simulink library "HDL_ieee_8021513"  (R2024a)
settings: Solver=FixedStepDiscrete  StartTime=0.0  StopTime=10.0  RelTol=1e-3
undefined symbols (not defined in the file): Add, axiWidth, CONST, fs, peakDetectorThreshold, peakDetectorWindow, QAM, Shift
libraries: hdlsllib x199, $bdroot x91, whdlutilities x34, whdledac x9, simulink x8, whdlmod x6, dspsigops x5, dsphdlfiltering2 x4, embreciprocals x3, dsphdlsigops2 x2, commhdlcrc x2, dspstat3 x2
(part 1 of 6)
settings Model: Creator=cotti  LastModifiedBy=cotti
settings OptimizationCC: BlockReduction=off  ConditionallyExecuteInputs=off  DefaultParameterBehavior=Inlined  InheritOutputTypeSmallerThanSingle=on  ReuseModelBlockBuffer=off
settings DebuggingCC: AlgebraicLoopMsg=error  SingleTaskRateTransMsg=error
settings HardwareCC: ProdBitPerPointer=32  ProdBitPerSizeT=32  ProdBitPerPtrDiffT=32  ProdLargestAtomicFloat=None  ProdIntDivRoundTo=Undefined  ProdEndianess=Unspecified  ProdWordSize=32  ProdHWDeviceType=ASIC/FPGA->ASIC/FPGA  TargetBitPerLong=64  TargetBitPerPointer=64  TargetBitPerSizeT=64  TargetBitPerPtrDiffT=64  TargetLongLongMode=on  TargetIntDivRoundTo=Zero  TargetEndianess=LittleEndian  TargetWordSize=64  TargetHWDeviceType=Custom Processor->MATLAB Host Computer  ProdEqTarget=off
settings RTWCC: GPUComputeCapability=3.5

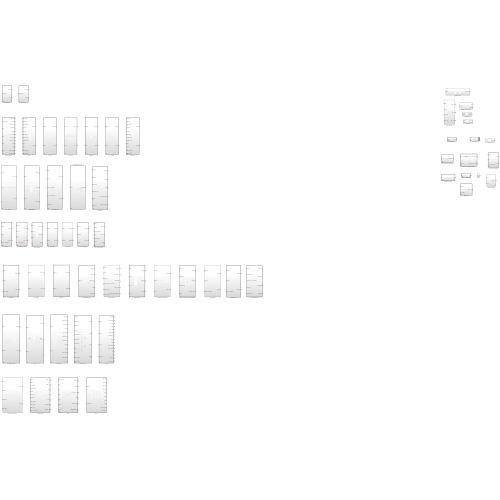
[thumbnail: Simulink's stored preview of the top-level diagram]
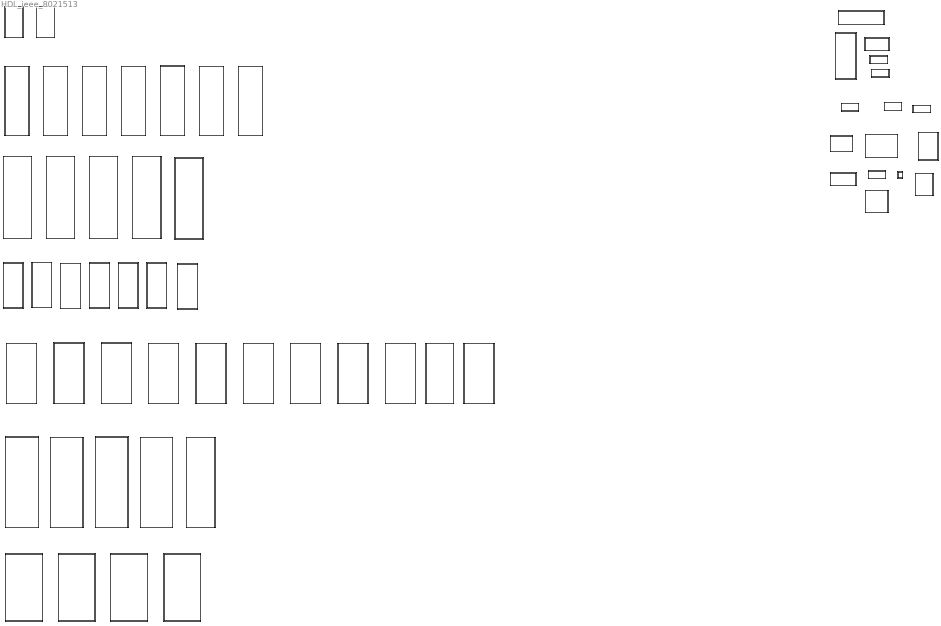
== system HDL_ieee_8021513 ==
  4QAM_demod : Subsystem  TreatAsAtomicUnit=on
  Buffer : Subsystem
  Deco_3a8 : Subsystem
  batid_to_bits_per_subcarrier : Subsystem
  calculate_mean_and_std : Subsystem
  channel_estimation_and_equalization : Subsystem  TreatAsAtomicUnit=on
  channel_gen : Subsystem
  complex_multiplier : Subsystem
  constellation_descrambler : Subsystem
  constellation_scrambler : Subsystem
  decimator : Subsystem  TreatAsAtomicUnit=on
  downshifter : Subsystem  TreatAsAtomicUnit=on
  falling_edge_detector : Subsystem
  frequency_upshift : Subsystem
  full_ofdm_modulator : Subsystem  TreatAsAtomicUnit=on
  full_rx : Subsystem  TreatAsAtomicUnit=on
  full_tx : Subsystem  TreatAsAtomicUnit=on
  gnd_ctrl : Subsystem
  h_crc : Subsystem
  h_crc_rx : Subsystem
  h_gen : Subsystem
  h_remove_repetition : Subsystem
  h_repetition : Subsystem
  h_rx_full : Subsystem  TreatAsAtomicUnit=on
  h_scrambler : Subsystem
      settings: LibrarySourceBlock=|
      | hdlsllib/Ports &
      | Subsystems/Subsystem
  h_separate : Subsystem
  header_fec : Subsystem
  header_full : Subsystem  TreatAsAtomicUnit=on
      settings: LibrarySourceBlock=|
      | hdlsllib/Ports &
      | Subsystems/Subsystem
  interpolator : Subsystem
  ldpc_encoder : Subsystem
  lfsr_const_scrambler : Subsystem
  next_frame_to_ready : Subsystem
  ofdm_demod : Subsystem  TreatAsAtomicUnit=on
  ofdm_modulator : Subsystem
  ofdm_separator : Subsystem
  ofdm_symbol_sync : Subsystem  TreatAsAtomicUnit=on
  p_scrambler : Subsystem
      settings: LibrarySourceBlock=|
      | hdlsllib/Ports &
      | Subsystems/Subsystem
  payload_full : Subsystem  TreatAsAtomicUnit=on
  payload_rep : Subsystem
  peak_detector : Subsystem
  preamble_gen : Subsystem
  psdu_size_to_payload_length : Subsystem
  puncturer : Subsystem
  qam_demod : Subsystem
  qam_mod : Subsystem
  reduced_ldpc : Subsystem
  reg_to_variable : Subsystem
  remove_tone_mapping : Subsystem
  rising_edge_detector : Subsystem
  rx_demodulator_full : Subsystem  TreatAsAtomicUnit=on
  rx_interpolator : Subsystem
  rx_payload_full : Subsystem  TreatAsAtomicUnit=on
  signal_ack : Subsystem
  tone_mapping : Subsystem
  tx_decimator : Subsystem
  valid_to_ctrl : Subsystem
  variable_to_reg : Subsystem

== system HDL_ieee_8021513/4QAM_demod ==
  data_in : Inport
  valid_in : Inport  Port=2
  bits_per_subcarrier : Inport  Port=3
  Delay{,1,3..4} (4 alike) : Delay  DelayLength=1  InitialCondition=0  UseCircularBuffer=on
  Delay2 : Delay  DelayLength=5  InitialCondition=0  UseCircularBuffer=on
  Symbol Demodulator1 : whdlmod/Symbol Demodulator  ModulationSource=Property  ModulationScheme=QPSK  MaxModulation=256-QAM  ConstOrder=Default  ConstMap=[ 2, 3, 1, 0, 6, 7, 5, 4, 14, 15, 13, 12, 10, 11, 9, 8 ]  DecisionType=Approximate log-likelihood ratio  PhaseOffset=-pi/4  OutputType=Vector  NormMethod=Unit average power  MinSymDistance=2  NoiseVariance=off  SimulateUsing=Code generation
  Terminator : Terminator
  Terminator2 : Terminator
  convert_with_rounding : DataTypeConversion  OutDataTypeStr=CONST.rxQAMDemodDataType  RndMeth=Round  SaturateOnIntegerOverflow=off
  data_out : Outport
  valid_out : Outport  Port=2  VectorParamsAs1DForOutWhenUnconnected=off
  wires:
  Delay4/1 -> Delay1/1
  Delay3/1 -> convert_with_rounding/1
  convert_with_rounding/1 -> Delay/1
  Symbol Demodulator1/2 -> Terminator2/1
  data_in/1 -> Symbol Demodulator1/1
  Symbol Demodulator1/1 -> Delay3/1
  valid_in/1 -> Symbol Demodulator1/2, Delay2/1
  Delay1/1 -> valid_out/1
  Delay/1 -> data_out/1
  bits_per_subcarrier/1 -> Terminator/1
  Delay2/1 -> Delay4/1

== system HDL_ieee_8021513/Buffer ==
  I : Inport
  O : Outport
  wires:
  I/1 -> O/1

== system HDL_ieee_8021513/Deco_3a8 ==
  in0 : Inport
  in1 : Inport  Port=2
  in2 : Inport  Port=3
  Logical Operator{,1..7} (8 alike) : Logic  Inputs=3  IconShape=distinctive  AllPortsSameDT=off  OutDataTypeStr=boolean
  Logical Operator{8..11,13..15,17,21..22,25,27} (12 alike) : Logic  Operator=NOT  IconShape=distinctive  AllPortsSameDT=off  OutDataTypeStr=boolean
  m0 : Outport
  m1 : Outport  Port=2
  m2 : Outport  Port=3
  m3 : Outport  Port=4
  m4 : Outport  Port=5
  m5 : Outport  Port=6
  m6 : Outport  Port=7
  m7 : Outport  Port=8
  wires:
  Logical Operator/1 -> m0/1
  Logical Operator1/1 -> m1/1
  Logical Operator2/1 -> m2/1
  Logical Operator3/1 -> m3/1
  Logical Operator4/1 -> m4/1
  Logical Operator5/1 -> m5/1
  Logical Operator6/1 -> m6/1
  Logical Operator7/1 -> m7/1
  in0/1 -> [in0]
  in1/1 -> [in1]
  in2/1 -> [in2]
  [in0] -> Logical Operator8/1
  [in1] -> Logical Operator9/1
  [in2] -> Logical Operator10/1
  Logical Operator8/1 -> Logical Operator/1
  Logical Operator9/1 -> Logical Operator/2
  Logical Operator10/1 -> Logical Operator/3
  [in1] -> Logical Operator13/1
  [in2] -> Logical Operator11/1
  [in2] -> Logical Operator14/1
  [in0] -> Logical Operator15/1
  [in1] -> Logical Operator2/2
  [in2] -> Logical Operator17/1
  [in0] -> Logical Operator3/1
  [in1] -> Logical Operator3/2
  [in2] -> Logical Operator4/3
  [in0] -> Logical Operator21/1
  [in1] -> Logical Operator22/1
  [in2] -> Logical Operator5/3
  [in0] -> Logical Operator5/1
  [in1] -> Logical Operator25/1
  [in2] -> Logical Operator6/3
  [in0] -> Logical Operator27/1
  [in1] -> Logical Operator6/2
  [in2] -> Logical Operator7/3
  [in0] -> Logical Operator7/1
  [in1] -> Logical Operator7/2
  [in0] -> Logical Operator1/1
  Logical Operator13/1 -> Logical Operator1/2
  Logical Operator11/1 -> Logical Operator1/3
  Logical Operator15/1 -> Logical Operator2/1
  Logical Operator14/1 -> Logical Operator2/3
  Logical Operator22/1 -> Logical Operator4/2
  Logical Operator21/1 -> Logical Operator4/1
  Logical Operator17/1 -> Logical Operator3/3
  Logical Operator27/1 -> Logical Operator6/1
  Logical Operator25/1 -> Logical Operator5/2

== system HDL_ieee_8021513/batid_to_bits_per_subcarrier ==
  note: De momento, el valor de BATID va a coincidir con el valor de la cantidad de bits por subcarrier.
  note: Remember that "bat_id" is LSB first.
  bat_id : Inport
  Bit Concat : hdlsllib/Logic and Bit Operations/Bit Concat  numInputs=4
  Demux : Demux  Outputs=5
  State Control : StateControl  StateControl=Synchronous
  Terminator : Terminator
  bits_per_subcarrier : Outport
  wires:
  bat_id/1 -> Demux/1
  Demux/3 -> [bat2]
  Demux/2 -> [bat1]
  Demux/4 -> [bat3]
  Demux/5 -> Terminator/1
  Demux/1 -> [bat0]
  Bit Concat/1 -> bits_per_subcarrier/1
  [bat3] -> Bit Concat/1
  [bat2] -> Bit Concat/2
  [bat1] -> Bit Concat/3
  [bat0] -> Bit Concat/4

== system HDL_ieee_8021513/calculate_mean_and_std ==
  data_in : Inport
  Delay{6..8,10..11} (5 alike) : Delay  DelayLength=1  InitialCondition=0  UseCircularBuffer=on
  Square : Math  Operator=square  SignedPower=on  RndMeth=Zero
  Subtract : Sum  Inputs=+-  OutDataTypeStr=Inherit: Same as first input
  calculate_mean_x : Subsystem
  calculate_mean_x_squared : Subsystem
  multiply by 2 : hdlsllib/Logic and Bit Operations/Bit Shift  mode=Shift Left Logical  N=1
  std : Outport
  mean : Outport  Port=2
  wires:
  Delay11/1 -> mean/1
  Subtract/1 -> Delay8/1
  Delay10/1 -> Delay11/1
  Square/1 -> Delay7/1
  Delay8/1 -> multiply by 2/1
  Delay6/1 -> Subtract/1
  calculate_mean_x/1(mean) -> Delay10/1, Square/1
  Delay7/1 -> Subtract/2
  calculate_mean_x_squared/1(mean_x_squared) -> Delay6/1
  data_in/1 -> calculate_mean_x/1(data_in), calculate_mean_x_squared/1(data_in)
  multiply by 2/1 -> std/1

== system HDL_ieee_8021513/channel_estimation_and_equalization ==
  note: Stores the estimate from Channel Estimation subsystem for each frame and perform channel equalization.
  note: Estimates the channel frequency response for each frame.
  data_in : Inport
  valid_data : Inport  Port=2
  valid_channel : Inport  Port=3
  reset : Inport  Port=4
  Channel Equalization : Subsystem
  Channel Estimation : Subsystem
  Delay{1..6,10..11,13..14} (10 alike) : Delay  DelayLength=1  InitialCondition=0
  Delay21 : Delay  InitialCondition=0
  Delay22 : Delay  InitialCondition=0
  data_out : Outport
  valid_out : Outport  Port=2
  channel_est_out : Outport  Port=3
  wires:
  reset/1 -> Channel Estimation/3(reset)
  Delay4/1 -> channel_est_out/1
  Channel Equalization/3(channel_est_out) -> Delay4/1
  Channel Estimation/1(channel_estimate) -> Delay13/1  "channelEstimates"
  Delay22/1 -> Delay11/1
  Delay21/1 -> Delay10/1
  valid_channel/1 -> Delay2/1
  data_in/1 -> Delay1/1
  valid_data/1 -> Delay3/1
  Delay2/1 -> Channel Estimation/2(valid_in)
  Channel Estimation/2(valid_estimate) -> Delay14/1  "channelEstimatesValid"
  Delay3/1 -> Delay22/1
  Delay1/1 -> Channel Estimation/1(data_in), Delay21/1
  Channel Equalization/2(valid_out) -> Delay6/1
  Channel Equalization/1(data_out) -> Delay5/1
  Delay10/1 -> Channel Equalization/1(data_in)
  Delay11/1 -> Channel Equalization/2(valid_data)
  Delay13/1 -> Channel Equalization/3(channel_estimate_in)
  Delay14/1 -> Channel Equalization/4(valid_channel_estimate)
  Delay6/1 -> valid_out/1
  Delay5/1 -> data_out/1

== system HDL_ieee_8021513/channel_gen ==
  new_frame : Inport
  Delay : Delay  DelayLength=1  InitialCondition=0  UseCircularBuffer=on
  Direct Lookup Table (n-D) : LookupNDDirect  NumberOfTableDimensions=1  Table=CONST.channelLUT  DiagnosticForOutOfRangeInput=Error  RemoveProtectionInput=on  TableDataTypeStr=boolean
  HDL Counter : hdlsllib/Sources/HDL Counter  CountType=Count limited  CountInit=0  CountStep=1  CountMax=length(CONST.channelLUT)-1  CountFromType=Initial value  CountFrom=0  CountResetPort=off  CountLoadPort=off  CountEnbPort=on  CountDirPort=off  CountHitOutputPort=on  CountDataType=Unsigned  CountWordLen=nextpow2(length(CONST.channelLUT))  CountFracLen=0  CountSampTime=1
  Logical Operator : Logic  Operator=NOT  IconShape=distinctive  AllPortsSameDT=off  OutDataTypeStr=boolean
  Logical Operator1 : Logic  Operator=OR  IconShape=distinctive  AllPortsSameDT=off  OutDataTypeStr=boolean
  State Control : StateControl  StateControl=Synchronous
  Unit Delay Enabled Synchronous : hdlsllib/Discrete/Unit Delay Enabled Synchronous  InitialCondition=0.0  SampleTime=-1
  valid_to_ctrl : $bdroot/valid_to_ctrl  SystemSampleTime=-1  VariantActivationTime=update diagram  AllowFlexibleInterface=on  Latency=0  AutoFrameSizeCalculation=off
  data_out : Outport
  ctrl_out : Outport  Port=2
  wires:
  Unit Delay Enabled Synchronous/1 -> HDL Counter/1, valid_to_ctrl/1
  HDL Counter/1 -> Direct Lookup Table (n-D)/1
  Logical Operator/1 -> Unit Delay Enabled Synchronous/1
  Direct Lookup Table (n-D)/1 -> Delay/1
  valid_to_ctrl/1 -> ctrl_out/1
  Delay/1 -> data_out/1
  new_frame/1 -> Logical Operator1/1
  HDL Counter/2 -> Logical Operator1/2, Logical Operator/1
  Logical Operator1/1 -> Unit Delay Enabled Synchronous/2

== system HDL_ieee_8021513/complex_multiplier ==
  in_a : Inport
  in_b : Inport  Port=2
  Add : Sum
  Add1 : Sum
  Add2 : Sum
  Complex to Real-Imag1 : ComplexToRealImag
  Complex to Real-Imag2 : ComplexToRealImag
  Delay{,1..3,10} (5 alike) : Delay  DelayLength=1  InitialCondition=0  UseCircularBuffer=on
  Delay{4..9,11,13..14} (9 alike) : Delay  InitialCondition=0  UseCircularBuffer=on
  Product : Product
  Product1 : Product
  Product2 : Product
  Real-Imag to Complex : RealImagToComplex
  Subtract : Sum  Inputs=+-
  Subtract1 : Sum  Inputs=+-
  a_times_b : Outport
  wires:
  [xr] -> Delay7/1
  [yi] -> Delay9/1
  [xi] -> Delay14/1
  [yi] -> Add/2
  [yr] -> Add/1
  [xi] -> Subtract1/2
  [xr] -> Subtract1/1
  [yi] -> Subtract/2
  [yr] -> Subtract/1
  in_a/1 -> Complex to Real-Imag1/1
  Complex to Real-Imag1/1 -> Delay/1
  in_b/1 -> Complex to Real-Imag2/1
  Complex to Real-Imag2/1 -> Delay2/1
  Complex to Real-Imag1/2 -> Delay1/1
  Complex to Real-Imag2/2 -> Delay3/1
  Delay10/1 -> a_times_b/1
  Subtract1/1 -> Delay4/1
  Subtract/1 -> Delay5/1
  Add/1 -> Delay6/1
  Delay4/1 -> Product/1
  Product/1 -> Delay8/1
  Delay/1 -> [xr]
  Delay1/1 -> [xi]
  Delay2/1 -> [yr]
  Delay3/1 -> [yi]
  Delay9/1 -> Product/2
  Delay5/1 -> Product1/1
  Delay7/1 -> Product1/2
  Product1/1 -> Delay11/1
  Add1/1 -> Real-Imag to Complex/1
  Real-Imag to Complex/1 -> Delay10/1
  Product2/1 -> Delay13/1
  Delay6/1 -> Product2/1
  Delay14/1 -> Product2/2
  Delay13/1 -> Add2/2
  Delay11/1 -> Add1/1
  Delay8/1 -> Add2/1, Add1/2
  Add2/1 -> Real-Imag to Complex/2

== system HDL_ieee_8021513/constellation_descrambler ==
  data_in : Inport
  valid_in : Inport  Port=2
  init : Inport  Port=3
  rising_edge_detector : $bdroot/rising_edge_detector  SystemSampleTime=-1  VariantActivationTime=update diagram  AllowFlexibleInterface=on  Latency=0  AutoFrameSizeCalculation=off
  rotate_-90 : Subsystem
  sync_constellation_scrambler : $bdroot/sync_constellation_scrambler  SystemSampleTime=-1  VariantActivationTime=update diagram  AllowFlexibleInterface=on  Latency=0  AutoFrameSizeCalculation=off
  data_out : Outport
  valid_out : Outport  Port=2
  wires:
  rising_edge_detector/1 -> sync_constellation_scrambler/3  "start"
  rotate_-90/1(data_out) -> data_out/1
  rotate_-90/2(valid_out) -> valid_out/1
  sync_constellation_scrambler/2 -> rotate_-90/4(s2_in)  "s2"
  sync_constellation_scrambler/1 -> rotate_-90/3(s1_in)  "s1"
  valid_in/1 -> rising_edge_detector/1, sync_constellation_scrambler/1, rotate_-90/2(valid_in)  "valid"
  init/1 -> sync_constellation_scrambler/2
  data_in/1 -> rotate_-90/1(data_in)

== system HDL_ieee_8021513/constellation_scrambler ==
  data_in : Inport
  valid_in : Inport  Port=2
  init : Inport  Port=3
  new_ofdm_symbol : Inport  Port=4
  Delay{,1..8} (9 alike) : Delay  DelayLength=1  InitialCondition=0  UseCircularBuffer=on
  Logical Operator : Logic  Operator=OR  IconShape=distinctive  AllPortsSameDT=off  OutDataTypeStr=boolean
  State Control : StateControl  StateControl=Synchronous
  lfsr_const_scrambler : $bdroot/lfsr_const_scrambler  SystemSampleTime=-1  VariantActivationTime=update diagram  AllowFlexibleInterface=on  Latency=0  AutoFrameSizeCalculation=off
  rotate : Subsystem
  data_out : Outport  VectorParamsAs1DForOutWhenUnconnected=off
  valid_out : Outport  Port=2  VectorParamsAs1DForOutWhenUnconnected=off
  wires:
  Delay1/1 -> rotate/2(valid_in)
  Delay/1 -> rotate/1(data_in)
  rotate/2(valid_out) -> Delay3/1
  Delay8/1 -> Delay1/1
  Delay4/1 -> rotate/3(s1)
  new_ofdm_symbol/1 -> lfsr_const_scrambler/3
  init/1 -> lfsr_const_scrambler/2
  Logical Operator/1 -> lfsr_const_scrambler/1
  Delay5/1 -> rotate/4(s2)
  Delay6/1 -> Logical Operator/2
  lfsr_const_scrambler/1 -> Delay4/1
  lfsr_const_scrambler/2 -> Delay5/1
  valid_in/1 -> Logical Operator/1, Delay6/1, Delay8/1  "en"
  data_in/1 -> Delay7/1
  Delay7/1 -> Delay/1  "data_in"
  rotate/1(data_out) -> Delay2/1  "data_out"
  Delay2/1 -> data_out/1  "data_out"
  Delay3/1 -> valid_out/1

== system HDL_ieee_8021513/decimator ==
  note: The data out from this blocks is "valid" one sample, and invalid four samples.
      | This blocks makes sure that the data is valid the five cycles.
      | What happens is that the ZOH might sample the signal when is valid or invalid.
  data_in : Inport
  valid_in : Inport  Port=2
  Delay{,1..2,5,8..11} (8 alike) : Delay  DelayLength=1  InitialCondition=0  UseCircularBuffer=on
  Delay3 : Delay  DelayLength=(CONST.rxDecimatorDelay+2)*3  InitialCondition=0  UseCircularBuffer=on
  Delay4 : Delay  DelayLength=CONST.rxDecimatorDelay/CONST.rxM  InitialCondition=0  UseCircularBuffer=on
  Downsample : DownSample  N=CONST.rxM  RateOptions=Allow multirate processing
  Downsample1 : DownSample  N=CONST.rxM  RateOptions=Allow multirate processing
  FIR Decimator : dsphdlfiltering2/FIR Decimator  Numerator=CONST.rxDecimatorFilter.Numerator  FilterStructure=Direct form systolic  DecimationFactor=CONST.rxM  NumCycles=1  SimulateUsing=Code generation  roundingMode=Floor  overflowMode=off  CoefficientsDataTypeStr=CONST.rxDecimatorCoefficientsDataType  OutputDataTypeStr=CONST.rxDecimatorOutputDataType  ResetInputPort=on  HDLGlobalReset=on
  Logical Operator : Logic  Operator=OR  IconShape=distinctive  AllPortsSameDT=off  OutDataTypeStr=boolean
  Logical Operator1 : Logic  Operator=OR  AllPortsSameDT=off  OutDataTypeStr=boolean
  Logical Operator2 : Logic  IconShape=distinctive  AllPortsSameDT=off  OutDataTypeStr=boolean
  Logical Operator3 : Logic  IconShape=distinctive  AllPortsSameDT=off  OutDataTypeStr=boolean
  Logical Operator4 : Logic  Operator=NOT  IconShape=distinctive  AllPortsSameDT=off  OutDataTypeStr=boolean
  Switch : Switch  Criteria=u2 ~= 0  SaturateOnIntegerOverflow=off  InputSameDT=off
  Unit Delay : UnitDelay  SampleTime=-1  HasFrameUpgradeWarning=on
  falling_edge_detector : $bdroot/falling_edge_detector  SystemSampleTime=-1  VariantActivationTime=update diagram  AllowFlexibleInterface=on  Latency=0  AutoFrameSizeCalculation=off
  rising_edge_detector : $bdroot/rising_edge_detector  SystemSampleTime=-1  VariantActivationTime=update diagram  AllowFlexibleInterface=on  Latency=0  AutoFrameSizeCalculation=off
  data_out : Outport
  valid_out : Outport  Port=2
  wires:
  Unit Delay/1 -> Switch/3
  Delay11/1 -> Logical Operator1/1
  Delay1/1 -> Logical Operator/1, Delay3/1
  Downsample1/1 -> Delay2/1  "data_after_down"
  Delay10/1 -> Delay5/1
  valid_in/1 -> Delay1/1, rising_edge_detector/1
  Delay3/1 -> Logical Operator/2
  falling_edge_detector/1 -> Logical Operator4/1
  FIR Decimator/1 -> Switch/1  "data_out"
  data_in/1 -> Delay10/1  "data_in"
  Delay9/1 -> data_out/1
  Delay5/1 -> FIR Decimator/1
  Logical Operator1/1 -> Downsample/1
  FIR Decimator/2 -> Switch/2, Delay11/1, Logical Operator1/2  "valid_out"
  Downsample/1 -> Delay8/1  "valid_after_down"
  Delay/1 -> Logical Operator3/1
  Delay4/1 -> Logical Operator2/2
  rising_edge_detector/1 -> FIR Decimator/3
  Logical Operator3/1 -> valid_out/1
  Delay2/1 -> Delay9/1
  Logical Operator4/1 -> Logical Operator3/2
  Logical Operator2/1 -> Delay/1, falling_edge_detector/1
  Logical Operator/1 -> FIR Decimator/2
  Delay8/1 -> Logical Operator2/1, Delay4/1
  Switch/1 -> Downsample1/1, Unit Delay/1

== system HDL_ieee_8021513/downshifter ==
  data_in : Inport
  valid_in : Inport  Port=2
  phase_offset : Inport  Port=3
  Add : Sum  OutDataTypeStr=Inherit: Same as first input
  Constant : Constant  Value=2^(CONST.ncoWordLength-2)  OutDataTypeStr=fixdt(0,CONST.ncoWordLength, 0)  SampleTime=1/CONST.fADC
  Constant1 : Constant  Value=fi(2^(CONST.ncoWordLength-1)/CONST.preambleFirstPartOFDMSamples, 0, CONST.rxFreqOffsetWordLength, CONST.rxFreqOffsetFractionLength)  OutDataTypeStr=fixdt(0, CONST.rxFreqOffsetWordLength, CONST.rxFreqOffsetFractionLength)  SampleTime=-1
  Delay : Delay  DelayLength=6  InitialCondition=0  UseCircularBuffer=on
  Delay1 : Delay  DelayLength=4  InitialCondition=0  UseCircularBuffer=on
  Delay{2..3,5,7..12} (9 alike) : Delay  InitialCondition=0  UseCircularBuffer=on
  Delay4 : Delay  DelayLength=1  InitialCondition=0  UseCircularBuffer=on
  NCO : dsphdlsigops2/NCO  PhaseIncrementSource=Input port  PhaseIncrement=ncoPhaseIncrement  PhaseOffsetSource=Property  PhaseOffset=0  DitherSource=None  NumDitherBits=1  SamplesPerFrame=1  LUTCompress=off  ResetAction=on  Waveform=Complex exponential  PhasePort=off  SimulateUsing=Code generation  AccumulatorWL=CONST.ncoWordLength  PhaseQuantization=on  NumQuantizerAccumulatorBits=CONST.ncoQuantization  OutputDataType=Binary point scaling  OutputWL=CONST.rxNCOWordLength  OutputFL=CONST.rxNCOFractionLength
  Product : Product  OutDataTypeStr=int16
  digital_carrier_receiver : Subsystem
  rising_edge_detector : $bdroot/rising_edge_detector  SystemSampleTime=-1  VariantActivationTime=update diagram  AllowFlexibleInterface=on  Latency=0  AutoFrameSizeCalculation=off
  data_out : Outport  VectorParamsAs1DForOutWhenUnconnected=off
  valid_out : Outport  Port=2  VectorParamsAs1DForOutWhenUnconnected=off
  wires:
  Constant1/1 -> Product/2
  Delay12/1 -> Delay7/1
  Delay11/1 -> Delay8/1
  Constant/1 -> Add/1
  Delay10/1 -> Add/2
  Delay9/1 -> Product/1
  Product/1 -> Delay10/1
  Delay4/1 -> rising_edge_detector/1
  valid_in/1 -> Delay12/1
  Delay1/1 -> valid_out/1
  NCO/2 -> Delay1/1
  Delay3/1 -> Delay/1
  digital_carrier_receiver/1(data_out) -> data_out/1
  NCO/1 -> digital_carrier_receiver/2(ncoIn)
  Delay/1 -> digital_carrier_receiver/1(dataIn)
  data_in/1 -> Delay11/1
  Delay2/1 -> NCO/3  "valid"
  rising_edge_detector/1 -> NCO/2
  Delay5/1 -> NCO/1  "inc"
  Add/1 -> Delay5/1
  Delay7/1 -> Delay2/1, Delay4/1
  Delay8/1 -> Delay3/1
  phase_offset/1 -> Delay9/1

== system HDL_ieee_8021513/falling_edge_detector ==
  in : Inport
  Delay : Delay  DelayLength=1  InitialCondition=0  UseCircularBuffer=on
  Logical Operator : Logic  IconShape=distinctive  AllPortsSameDT=off  OutDataTypeStr=boolean
  Logical Operator1 : Logic  Operator=NOT  IconShape=distinctive  AllPortsSameDT=off  OutDataTypeStr=boolean
  State Control : StateControl  StateControl=Synchronous
  out : Outport  VectorParamsAs1DForOutWhenUnconnected=off
  wires:
  in/1 -> Logical Operator1/1, Delay/1
  Delay/1 -> Logical Operator/2
  Logical Operator/1 -> out/1
  Logical Operator1/1 -> Logical Operator/1

== system HDL_ieee_8021513/frequency_upshift ==
  data_in : Inport
  valid_in : Inport  Port=2
  reset : Inport  Port=3
  Data Type Conversion : DataTypeConversion  OutDataTypeStr=CONST.ipCoreDataType  SaturateOnIntegerOverflow=off  RndMeth=Floor
  Delay : Delay  DelayLength=6  InitialCondition=0  UseCircularBuffer=on
  Delay1 : Delay  DelayLength=12  InitialCondition=0  UseCircularBuffer=on
  Delay2 : Delay  DelayLength=1  InitialCondition=0  UseCircularBuffer=on
  Delay3 : Delay  DelayLength=1  InitialCondition=0  UseCircularBuffer=on
  Mixer : Subsystem
  NCO : dsphdlsigops2/NCO  PhaseIncrementSource=Property  PhaseIncrement=CONST.ncoUpCarrierPhaseIncrement  PhaseOffsetSource=Property  PhaseOffset=0  DitherSource=None  NumDitherBits=1  SamplesPerFrame=1  LUTCompress=off  ResetAction=on  Waveform=Complex exponential  PhasePort=off  SimulateUsing=Code generation  AccumulatorWL=CONST.ncoUpWordLength  PhaseQuantization=on  NumQuantizerAccumulatorBits=CONST.ncoUpQuantization  OutputDataType=Binary point scaling  OutputWL=CONST.txNCOWordLength  OutputFL=CONST.txNCOFractionLength
  State Control : StateControl  StateControl=Synchronous
  data_out : Outport  VectorParamsAs1DForOutWhenUnconnected=off
  valid_out : Outport  Port=2  VectorParamsAs1DForOutWhenUnconnected=off
  wires:
  Data Type Conversion/1 -> data_out/1
  Delay2/1 -> NCO/2
  reset/1 -> NCO/1
  Delay3/1 -> Delay/1
  data_in/1 -> Delay3/1
  valid_in/1 -> Delay2/1
  NCO/1 -> Mixer/2(ncoIn)
  Mixer/1(mixedOut) -> Data Type Conversion/1
  Delay/1 -> Mixer/1(dataIn)
  NCO/2 -> Delay1/1
  Delay1/1 -> valid_out/1

== system HDL_ieee_8021513/full_ofdm_modulator ==
  data_in : Inport
  valid_in : Inport  Port=2
  bits_per_subcarrier : Inport  Port=3
  init : Inport  Port=4
  new_ofdm_sym : Inport  Port=5
  cp_len : Inport  Port=6
  rst : Inport  Port=7
  Constant : Constant  Value=0  OutDataTypeStr=fixdt(1,16,14)  SampleTime=-1
  Delay{,1,4..11} (10 alike) : Delay  DelayLength=1  InitialCondition=0  UseCircularBuffer=on
  HDL FIFO : hdlsllib/HDL RAMs/HDL FIFO  fifo_size=CONST.preambleFirstPartOFDMSamples  mode=Classic  ratio=1  push_msg=Error  pop_msg=Error  show_empty=on  show_full=on  show_num=off  LabelModeActiveChoice_Mode=Classic  rst_port=on
  Logical Operator1 : Logic  Operator=OR  AllPortsSameDT=off  OutDataTypeStr=boolean
  Real-Imag to Complex : RealImagToComplex
  Repeat : dspsigops/Repeat  FactorSource=Dialog parameter  N=CONST.txL  Nmax=16  RateOptions=Allow multirate processing  ic=0  mode=Unused parameter value
      settings: LibrarySourceBlock=dsphdlsupportsigops/Repeat
  State Control : StateControl  StateControl=Synchronous
  Switch : Switch  Criteria=u2 ~= 0  SaturateOnIntegerOverflow=off  InputSameDT=off
  Switch1 : Switch  Criteria=u2 ~= 0  SaturateOnIntegerOverflow=off  InputSameDT=off
  Unit Delay : UnitDelay  SampleTime=-1  HasFrameUpgradeWarning=on
  constellation_scrambler : $bdroot/constellation_scrambler  SystemSampleTime=-1  VariantActivationTime=update diagram  AllowFlexibleInterface=on  Latency=0  AutoFrameSizeCalculation=off
  frequency_upshift : $bdroot/frequency_upshift  SystemSampleTime=-1  VariantActivationTime=update diagram  AllowFlexibleInterface=on  Latency=0  AutoFrameSizeCalculation=off
  interpolator : $bdroot/interpolator  SystemSampleTime=-1  VariantActivationTime=update diagram  AllowFlexibleInterface=on  Latency=0  AutoFrameSizeCalculation=off
  ofdm_modulator : $bdroot/ofdm_modulator  SystemSampleTime=-1  VariantActivationTime=update diagram  AllowFlexibleInterface=on  Latency=0  AutoFrameSizeCalculation=off
  ofdm_ready_truncate : Subsystem
  qam_mod : $bdroot/qam_mod  SystemSampleTime=-1  VariantActivationTime=update diagram  AllowFlexibleInterface=on  Latency=0  AutoFrameSizeCalculation=off
  data_out : Outport  VectorParamsAs1DForOutWhenUnconnected=off
  valid_out : Outport  Port=2  VectorParamsAs1DForOutWhenUnconnected=off
  ready : Outport  Port=3  VectorParamsAs1DForOutWhenUnconnected=off
  wires:
  Constant/1 -> Real-Imag to Complex/1, Real-Imag to Complex/2
  Real-Imag to Complex/1 -> Switch1/3
  HDL FIFO/1 -> Switch1/1  "fifo_out"
  Switch1/1 -> interpolator/1
  ofdm_modulator/3 -> ofdm_ready_truncate/1(next_frame)  "ready_out"
  Delay10/1 -> qam_mod/2  "real_valid"
  Delay11/1 -> qam_mod/1
  Delay9/1 -> qam_mod/3
  Delay8/1 -> Delay/1
  Delay7/1 -> Delay1/1
  Delay5/1 -> ofdm_modulator/4, HDL FIFO/4, Repeat/1, ofdm_ready_truncate/2(new_psdu)  "fifo_rst"
  ofdm_ready_truncate/1(ready) -> ready/1  "ready"
  Repeat/1 -> frequency_upshift/3
  Delay4/1 -> interpolator/2, Switch1/2
  HDL FIFO/2 -> Logical Operator1/2  "fifo_empty"
  Logical Operator1/1 -> Switch/2
  Switch/1 -> HDL FIFO/3, Unit Delay/1, Delay4/1
  HDL FIFO/3 -> Logical Operator1/1, Switch/1
  Unit Delay/1 -> Switch/3
  ofdm_modulator/1 -> HDL FIFO/1
  ofdm_modulator/2 -> HDL FIFO/2
  rst/1 -> Delay5/1
  Delay1/1 -> constellation_scrambler/4
  Delay/1 -> constellation_scrambler/3
  qam_mod/2 -> constellation_scrambler/2
  qam_mod/1 -> constellation_scrambler/1
  new_ofdm_sym/1 -> Delay7/1
  constellation_scrambler/1 -> ofdm_modulator/1  "out_new"
  constellation_scrambler/2 -> ofdm_modulator/2  "valid_new"
  data_in/1 -> Delay11/1
  valid_in/1 -> Delay10/1
  bits_per_subcarrier/1 -> Delay9/1
  init/1 -> Delay8/1
  cp_len/1 -> Delay6/1
  Delay6/1 -> ofdm_modulator/3
  interpolator/2 -> frequency_upshift/2
  interpolator/1 -> frequency_upshift/1
  frequency_upshift/2 -> valid_out/1
  frequency_upshift/1 -> data_out/1

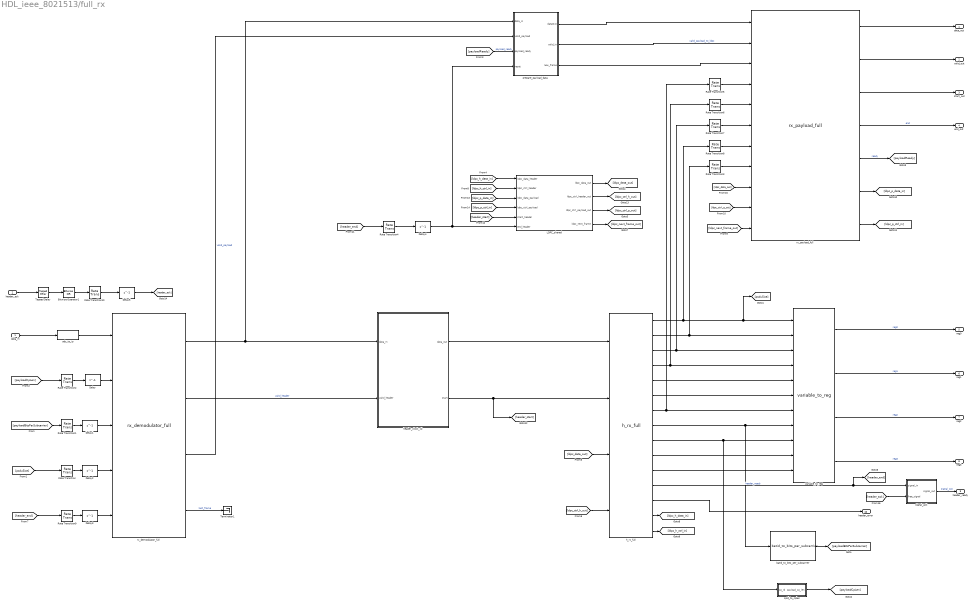
== system HDL_ieee_8021513/full_rx ==
  data_in : Inport
  header_ack : Inport  Port=2
  Bitwise Operator1 : simulink/Logic and Bit Operations/Bitwise Operator  logicop=OR  UseBitMask=off  BitMask=bin2dec('11011001')  BitMaskRealWorld=Stored Integer
      settings: LibrarySourceBlock=|
      | hdlsllib/Logic and Bit
      | Operations/Bitwise
      | Operator
  Delay{,1..5} (6 alike) : Delay  DelayLength=1  InitialCondition=0  UseCircularBuffer=on
  LDPC_shared : Subsystem
  Rate Transition{,1..2,9} (4 alike) : RateTransition  OutPortSampleTime=1/CONST.fPHY
  Rate Transition10 : RateTransition  OutPortSampleTimeOpt=Multiple of input port sample time  OutPortSampleTimeMultiple=8
  Rate Transition{3,5..8} (5 alike) : RateTransition  OutPortSampleTime=1/CONST.fs
  Rate Transition4 : RateTransition  OutPortSampleTimeOpt=Multiple of input port sample time  OutPortSampleTimeMultiple=1/8
  Tapped Delay : simulink/Discrete/Tapped Delay  vinit=0.0  samptime=-1  NumDelays=8  DelayOrder=Oldest  includeCurrent=off
      settings: LibrarySourceBlock=hdlsllib/Discrete/Tapped Delay
  Terminator1 : Terminator
  adc_to_ip : DataTypeConversion  OutDataTypeStr=CONST.ADCDataType  ConvertRealWorld=Stored Integer (SI)  SaturateOnIntegerOverflow=off  RndMeth=Floor
  batid_to_bits_per_subcarrier : $bdroot/batid_to_bits_per_subcarrier  SystemSampleTime=-1  VariantActivationTime=update diagram  AllowFlexibleInterface=on  Latency=0  AutoFrameSizeCalculation=off
  cpid_to_cplen : Subsystem
  h_rx_full : $bdroot/h_rx_full  SystemSampleTime=-1  VariantActivationTime=update diagram  AllowFlexibleInterface=on  Latency=0  AutoFrameSizeCalculation=off
  header_clock_x2 : Subsystem
  prepare_payload_data : Subsystem
  rx_demodulator_full : $bdroot/rx_demodulator_full  SystemSampleTime=-1  VariantActivationTime=update diagram  AllowFlexibleInterface=on  Latency=0  AutoFrameSizeCalculation=off
  rx_payload_full : $bdroot/rx_payload_full  SystemSampleTime=-1  VariantActivationTime=update diagram  AllowFlexibleInterface=on  Latency=0  AutoFrameSizeCalculation=off
  signal_ack : Subsystem
  variable_to_reg : $bdroot/variable_to_reg  SystemSampleTime=-1  VariantActivationTime=update diagram  AllowFlexibleInterface=on  Latency=0  AutoFrameSizeCalculation=off
  data_out : Outport
  valid_out : Outport  Port=2
  start_out : Outport  Port=3
  end_out : Outport  Port=4
  reg0 : Outport  Port=5
  reg1 : Outport  Port=6
  reg2 : Outport  Port=7
  reg3 : Outport  Port=8
  header_ready : Outport  Port=9
  header_error : Outport  Port=10
  wires:
  [header_ack] -> signal_ack/2(free_signal)
  signal_ack/1(signal_out) -> header_ready/1  "signal_out"
  Delay5/1 -> [header_ack]
  Bitwise Operator1/1 -> Rate Transition10/1
  Rate Transition10/1 -> Delay5/1
  Tapped Delay/1 -> Bitwise Operator1/1
  header_ack/1 -> Tapped Delay/1
  adc_to_ip/1 -> rx_demodulator_full/1
  Delay4/1 -> LDPC_shared/6(end_header), prepare_payload_data/4(reset)
  [header_end] -> Rate Transition4/1
  Rate Transition4/1 -> Delay4/1
  [ldpc_data_out] -> rx_payload_full/9
  [ldpc_ctrl_p_out] -> rx_payload_full/10
  LDPC_shared/2(ldpc_ctrl_header_out) -> [ldpc_ctrl_h_out]
  LDPC_shared/3(ldpc_ctrl_payload_out) -> [ldpc_ctrl_p_out]
  [ldpc_h_ctrl_in] -> LDPC_shared/2(ldpc_ctrl_header)
  [ldpc_p_ctrl_in] -> LDPC_shared/4(ldpc_ctrl_payload)
  [ldpc_h_data_in] -> LDPC_shared/1(ldpc_data_header)
  [ldpc_p_data_in] -> LDPC_shared/3(ldpc_data_payload)
  [header_start] -> LDPC_shared/5(start_header)
  LDPC_shared/4(ldpc_next_frame) -> [ldpc_next_frame_out]
  LDPC_shared/1(ldpc_data_out) -> [ldpc_data_out]
  rx_payload_full/7 -> [ldpc_p_ctrl_in]
  rx_payload_full/6 -> [ldpc_p_data_in]
  [ldpc_next_frame_out] -> rx_payload_full/11
  [ldpc_ctrl_h_out] -> h_rx_full/4
  [ldpc_data_out] -> h_rx_full/3
  h_rx_full/15 -> [ldpc_h_ctrl_in]
  h_rx_full/14 -> [ldpc_h_data_in]
  rx_payload_full/4 -> end_out/1  "end"
  rx_payload_full/3 -> start_out/1
  Rate Transition3/1 -> rx_payload_full/8
  prepare_payload_data/3(new_frame) -> rx_payload_full/3
  rx_payload_full/5 -> [payloadReady]  "ready"
  Delay3/1 -> rx_demodulator_full/5
  Delay2/1 -> rx_demodulator_full/4
  Delay1/1 -> rx_demodulator_full/3
  Delay/1 -> rx_demodulator_full/2
  rx_demodulator_full/3 -> prepare_payload_data/2(valid_payload)  "valid_payload"
  rx_demodulator_full/2 -> header_clock_x2/2(valid_header)  "valid_header"
  Rate Transition9/1 -> Delay3/1
  Rate Transition/1 -> Delay2/1
  Rate Transition1/1 -> Delay1/1
  Rate Transition2/1 -> Delay/1
  h_rx_full/6 -> variable_to_reg/6
  batid_to_bits_per_subcarrier/1 -> [payloadBitsPerSubcarrier]
  Rate Transition7/1 -> rx_payload_full/6
  variable_to_reg/1 -> reg0/1  "reg0"
  header_clock_x2/2(start) -> h_rx_full/2, [header_start]
  cpid_to_cplen/1(payload_cp_len) -> [payloadCpLen]
  h_rx_full/10 -> variable_to_reg/10
  Rate Transition5/1 -> rx_payload_full/4
  Rate Transition6/1 -> rx_payload_full/5
  h_rx_full/5 -> variable_to_reg/5
  data_in/1 -> adc_to_ip/1
  h_rx_full/4 -> Rate Transition6/1, variable_to_reg/4
  prepare_payload_data/1(dataOut) -> rx_payload_full/1
  h_rx_full/3 -> Rate Transition7/1, variable_to_reg/3
  rx_demodulator_full/1 -> header_clock_x2/1(data_in), prepare_payload_data/1(data_in)
  Rate Transition8/1 -> rx_payload_full/7
  h_rx_full/11 -> variable_to_reg/11
  [payloadReady] -> prepare_payload_data/3(payload_ready)  "payload_ready"
  rx_payload_full/1 -> data_out/1
  h_rx_full/8 -> batid_to_bits_per_subcarrier/1, variable_to_reg/8
  rx_payload_full/2 -> valid_out/1
  h_rx_full/1 -> Rate Transition8/1, [psduSize], variable_to_reg/1
  h_rx_full/2 -> variable_to_reg/2, Rate Transition3/1
  h_rx_full/9 -> variable_to_reg/9, cpid_to_cplen/1(cp_id)
  prepare_payload_data/2(valid_in) -> rx_payload_full/2  "valid_payload_to_ldpc"
  [psduSize] -> Rate Transition/1
  [payloadCpLen] -> Rate Transition2/1
  h_rx_full/13 -> header_error/1
  h_rx_full/7 -> Rate Transition5/1, variable_to_reg/7
  [payloadBitsPerSubcarrier] -> Rate Transition1/1
  header_clock_x2/1(data_out) -> h_rx_full/1
  variable_to_reg/4 -> reg3/1  "reg3"
  variable_to_reg/2 -> reg1/1  "reg1"
  variable_to_reg/3 -> reg2/1  "reg2"
  h_rx_full/12 -> [header_end], signal_ack/1(signal_in)  "header_ready"
  [header_end] -> Rate Transition9/1
  rx_demodulator_full/4 -> Terminator1/1  "last_frame"

== system HDL_ieee_8021513/full_tx ==
  new_frame_in : Inport
  reg0 : Inport  Port=2
  reg1 : Inport  Port=3
  reg2 : Inport  Port=4
  reg3 : Inport  Port=5
  data_in : Inport  Port=6
  valid_in : Inport  Port=7
  Delay{10..17} (8 alike) : Delay  DelayLength=8  InitialCondition=0  UseCircularBuffer=on
  Delay7 : Delay  DelayLength=1  InitialCondition=0  UseCircularBuffer=on
  Delay8 : Delay  DelayLength=1  InitialCondition=0  UseCircularBuffer=on
  Delay9 : Delay  DelayLength=1  InitialCondition=0  UseCircularBuffer=on
  Rate Transition : RateTransition  OutPortSampleTime=1/CONST.fPHY
  Rate Transition1 : RateTransition  OutPortSampleTime=1/CONST.fDAC
  Sample Control Bus Selector : whdlutilities/Sample Control Bus Selector  OutputSignals=start,end,valid
  State Control : StateControl  StateControl=Synchronous
  Terminator : Terminator
  Terminator1 : Terminator
  channel_gen : $bdroot/channel_gen  SystemSampleTime=-1  VariantActivationTime=update diagram  AllowFlexibleInterface=on  Latency=0  AutoFrameSizeCalculation=off
  clock_crossing : Subsystem
  falling_edge_detector : $bdroot/falling_edge_detector  SystemSampleTime=-1  VariantActivationTime=update diagram  AllowFlexibleInterface=on  Latency=0  AutoFrameSizeCalculation=off
  full_ofdm_modulator : $bdroot/full_ofdm_modulator  SystemSampleTime=-1  VariantActivationTime=update diagram  AllowFlexibleInterface=on  Latency=0  AutoFrameSizeCalculation=off
  header_full : $bdroot/header_full  SystemSampleTime=-1  VariantActivationTime=update diagram  AllowFlexibleInterface=on  Latency=0  AutoFrameSizeCalculation=off
      settings: LibrarySourceBlock=|
      | hdlsllib/Ports &
      | Subsystems/Subsystem
  ip_to_dac : DataTypeConversion  OutDataTypeStr=int16  ConvertRealWorld=Stored Integer (SI)  SaturateOnIntegerOverflow=off  RndMeth=Floor
  new_frame_rate_conversion : Subsystem
  new_frame_rate_conversion1 : Subsystem
  payload_full : $bdroot/payload_full  SystemSampleTime=-1  VariantActivationTime=update diagram  AllowFlexibleInterface=on  Latency=0  AutoFrameSizeCalculation=off
  preamble_gen : $bdroot/preamble_gen  SystemSampleTime=-1  VariantActivationTime=update diagram  AllowFlexibleInterface=on  Latency=0  AutoFrameSizeCalculation=off
  reg_to_variable : $bdroot/reg_to_variable  SystemSampleTime=-1  VariantActivationTime=update diagram  AllowFlexibleInterface=on  Latency=0  AutoFrameSizeCalculation=off
  rising_edge_detector : $bdroot/rising_edge_detector  SystemSampleTime=-1  VariantActivationTime=update diagram  AllowFlexibleInterface=on  Latency=0  AutoFrameSizeCalculation=off
  signal_ack : $bdroot/signal_ack  SystemSampleTime=-1  VariantActivationTime=update diagram  AllowFlexibleInterface=on  Latency=0  AutoFrameSizeCalculation=off
  store_frame_in_ram : Subsystem
  data_out : Outport
  valid_out : Outport  Port=2
  new_msg_ready : Outport  Port=3  VectorParamsAs1DForOutWhenUnconnected=off
  ready : Outport  Port=4
  debug_payload : Outport  Port=5  VectorParamsAs1DForOutWhenUnconnected=off
  debug_payload_ctrl : Outport  Port=6  VectorParamsAs1DForOutWhenUnconnected=off
  wires:
  store_frame_in_ram/7(new_psdu) -> full_ofdm_modulator/7  "new_psdu"
  Rate Transition1/1 -> signal_ack/2
  ip_to_dac/1 -> data_out/1
  full_ofdm_modulator/1 -> ip_to_dac/1
  falling_edge_detector/1 -> signal_ack/1  "b"
  [new_frame_rised] -> Rate Transition1/1
  signal_ack/1 -> new_msg_ready/1  "signal_out"
  rising_edge_detector/1 -> reg_to_variable/1, [new_frame_rised]  "new_frame_rised"
  new_frame_rate_conversion1/1(new_frame) -> payload_full/3  "payload_new_frame_in"
  Delay9/1 -> store_frame_in_ram/9(payload_len)
  Delay17/1 -> store_frame_in_ram/1(preamble)
  Delay16/1 -> store_frame_in_ram/2(preamble_valid)
  Delay15/1 -> store_frame_in_ram/3(channel)
  Delay14/1 -> store_frame_in_ram/4(channel_valid)
  Delay13/1 -> store_frame_in_ram/5(header)
  Delay12/1 -> store_frame_in_ram/6(header_valid)
  Delay11/1 -> store_frame_in_ram/7(payload)
  Delay10/1 -> store_frame_in_ram/8(payload_valid)
  Delay8/1 -> store_frame_in_ram/10(bits_per_subcarrier)
  Delay7/1 -> store_frame_in_ram/11(cp_len_in)
  store_frame_in_ram/1(data_out) -> full_ofdm_modulator/1
  store_frame_in_ram/2(valid_out) -> full_ofdm_modulator/2
  store_frame_in_ram/3(bits_per_subcarrier_out) -> full_ofdm_modulator/3
  store_frame_in_ram/4(init) -> full_ofdm_modulator/4
  store_frame_in_ram/5(new) -> full_ofdm_modulator/5
  store_frame_in_ram/6(cp_len) -> full_ofdm_modulator/6
  full_ofdm_modulator/3 -> store_frame_in_ram/12(ready)  "ofdm_ready"
  clock_crossing/1(preamble_out) -> Delay17/1
  clock_crossing/2(preamble_valid) -> Delay16/1
  clock_crossing/3(channel_out) -> Delay15/1
  clock_crossing/4(channel_valid) -> Delay14/1
  clock_crossing/5(header_out) -> Delay13/1
  clock_crossing/6(header_valid) -> Delay12/1
  clock_crossing/7(payload_out) -> Delay11/1
  clock_crossing/8(payload_valid_out) -> Delay10/1
  clock_crossing/9(payload_len_out) -> Delay9/1
  clock_crossing/10(bits_per_subcarrier_out) -> Delay8/1
  clock_crossing/11(cp_len_out) -> Delay7/1
  Sample Control Bus Selector/2 -> channel_gen/1  "<end>"
  Sample Control Bus Selector/3 -> Terminator/1  "<valid>"
  payload_full/1 -> clock_crossing/7(payload_in), debug_payload/1
  reg_to_variable/3 -> header_full/3
  channel_gen/2 -> new_frame_rate_conversion/1(ctrl_in), clock_crossing/4(channel_ctrl)
  payload_full/5 -> clock_crossing/11(bits_per_subcarrier_in)
  reg_to_variable/9 -> header_full/9, payload_full/5
  reg_to_variable/11 -> header_full/11
  header_full/2 -> new_frame_rate_conversion1/1(ctrl_in), clock_crossing/6(header_ctrl_in)
  Rate Transition/1 -> preamble_gen/1
  header_full/1 -> clock_crossing/5(header_in)
  reg_to_variable/8 -> header_full/8, payload_full/4
  reg_to_variable/10 -> clock_crossing/9(cp_len_in), header_full/10
  reg_to_variable/6 -> header_full/6
  valid_in/1 -> payload_full/2
  channel_gen/1 -> clock_crossing/3(channel)
  new_frame_in/1 -> rising_edge_detector/1
  new_frame_rate_conversion/1(new_frame) -> header_full/1
  preamble_gen/1 -> clock_crossing/1(preamble_in)
  reg1/1 -> reg_to_variable/3
  full_ofdm_modulator/2 -> valid_out/1, falling_edge_detector/1  "valid_out"
  reg3/1 -> reg_to_variable/5
  preamble_gen/2 -> clock_crossing/2(preamble_ctrl_in), Sample Control Bus Selector/1
  reg_to_variable/12 -> header_full/12
  reg2/1 -> reg_to_variable/4
  reg_to_variable/2 -> header_full/2, payload_full/6
  reg_to_variable/5 -> header_full/5
  payload_full/3 -> ready/1
  payload_full/4 -> clock_crossing/10(payload_len_in)
  reg_to_variable/1 -> Rate Transition/1
  reg_to_variable/7 -> header_full/7
  data_in/1 -> payload_full/1
  Sample Control Bus Selector/1 -> Terminator1/1  "<start>"
  reg0/1 -> reg_to_variable/2
  payload_full/2 -> clock_crossing/8(payload_ctrl_in), debug_payload_ctrl/1  "payload_ctrl_out"
  reg_to_variable/4 -> header_full/4

== system HDL_ieee_8021513/gnd_ctrl ==
  Ground : Ground
  Ground1 : Ground
  Ground2 : Ground
  Sample Control Bus Creator : whdlutilities/Sample Control Bus Creator
  gnd_ctrl : Outport
  wires:
  Ground/1 -> Sample Control Bus Creator/3
  Ground1/1 -> Sample Control Bus Creator/2
  Ground2/1 -> Sample Control Bus Creator/1
  Sample Control Bus Creator/1 -> gnd_ctrl/1

== system HDL_ieee_8021513/h_crc ==
  data_in : Inport
  ctrl_in : Inport  Port=2
  Delay{,1..3} (4 alike) : Delay  DelayLength=1  InitialCondition=0  UseCircularBuffer=on
  General CRC Generator HDL Optimized : commhdlcrc/General CRC Generator HDL Optimized  Polynomial=CONST.headerCRCPoly  InitialState=1  DirectMethod=on  ReflectInput=off  ReflectCRCChecksum=off  FinalXORValue=0  SimulateUsing=Code generation
  Sample Control Bus Creator : whdlutilities/Sample Control Bus Creator
  Sample Control Bus Selector : whdlutilities/Sample Control Bus Selector  OutputSignals=start,end,valid
  State Control : StateControl  StateControl=Synchronous
  data_out : Outport
  ctrl_out : Outport  Port=2
  wires:
  Delay3/1 -> Sample Control Bus Selector/1
  Delay2/1 -> General CRC Generator HDL Optimized/1
  Delay1/1 -> ctrl_out/1
  Delay/1 -> data_out/1
  Sample Control Bus Creator/1 -> Delay1/1
  General CRC Generator HDL Optimized/2 -> Sample Control Bus Creator/1
  General CRC Generator HDL Optimized/3 -> Sample Control Bus Creator/2
  General CRC Generator HDL Optimized/4 -> Sample Control Bus Creator/3
  General CRC Generator HDL Optimized/1 -> Delay/1
  data_in/1 -> Delay2/1
  ctrl_in/1 -> Delay3/1
  Sample Control Bus Selector/1 -> General CRC Generator HDL Optimized/2
  Sample Control Bus Selector/2 -> General CRC Generator HDL Optimized/3
  Sample Control Bus Selector/3 -> General CRC Generator HDL Optimized/4

== system HDL_ieee_8021513/h_crc_rx ==
  data_in : Inport
  ctrl_in : Inport  Port=2
  General CRC Syndrome Detector HDL Optimized : commhdlcrc/General CRC Syndrome Detector HDL Optimized  Polynomial=CONST.headerCRCPoly  InitialState=1  DirectMethod=on  ReflectInput=off  ReflectCRCChecksum=off  FinalXORValue=0  SimulateUsing=Code generation
  Sample Control Bus Creator : whdlutilities/Sample Control Bus Creator
  Sample Control Bus Selector : whdlutilities/Sample Control Bus Selector  OutputSignals=start,end,valid
  State Control : StateControl  StateControl=Synchronous
  Switch : Switch  Criteria=u2 ~= 0  SaturateOnIntegerOverflow=off  InputSameDT=off
  Unit Delay : UnitDelay  SampleTime=-1  HasFrameUpgradeWarning=on
  data_out : Outport
  ctrl_out : Outport  Port=2  VectorParamsAs1DForOutWhenUnconnected=off
  err : Outport  Port=3  VectorParamsAs1DForOutWhenUnconnected=off
  wires:
  ctrl_in/1 -> Sample Control Bus Selector/1
  Sample Control Bus Selector/3 -> General CRC Syndrome Detector HDL Optimized/4  "<valid>"
  Sample Control Bus Selector/2 -> General CRC Syndrome Detector HDL Optimized/3  "<end>"
  Sample Control Bus Selector/1 -> General CRC Syndrome Detector HDL Optimized/2  "<start>"
  data_in/1 -> General CRC Syndrome Detector HDL Optimized/1
  General CRC Syndrome Detector HDL Optimized/1 -> data_out/1
  General CRC Syndrome Detector HDL Optimized/2 -> Sample Control Bus Creator/1
  General CRC Syndrome Detector HDL Optimized/3 -> Switch/2, Sample Control Bus Creator/2
  General CRC Syndrome Detector HDL Optimized/4 -> Sample Control Bus Creator/3
  Sample Control Bus Creator/1 -> ctrl_out/1
  Unit Delay/1 -> Switch/3
  Switch/1 -> err/1, Unit Delay/1
  General CRC Syndrome Detector HDL Optimized/5 -> Switch/1
